simulink model "Vehicle_Model_Controller_Aug13"  (R2021b)
settings: Solver=VariableStepAuto  StartTime=0.0  StopTime=15  FixedStep=0.015  MaxStep=0.015  RelTol=1e-3
model workspace (MAT data in the model file):
  Cx = 10000
  Dx = 2000
  Kp = 10
  understeer_gradient = 0.05
values from neighbouring files (symbols this model uses):
  a = Simulink.Parameter(1.14)    [startup.m]
  A1 = Simulink.Parameter(39.8344)    [startup.m]
  A2 = Simulink.Parameter(813.0780)    [startup.m]
  b = Simulink.Parameter(-0.03291)    [startup.m]
  B1 = Simulink.Parameter(0.000001287)    [startup.m]
  B2 = Simulink.Parameter(-0.002325)    [startup.m]
  B3 = Simulink.Parameter(3.797)    [startup.m]
  c = Simulink.Parameter(-1.14)    [startup.m]
  C1 = Simulink.Parameter(-0.000000002541)    [startup.m]
  C2 = Simulink.Parameter(0.000005279)    [startup.m]
  C3 = Simulink.Parameter(-0.003943)    [startup.m]
  C4 = Simulink.Parameter(3.634)    [startup.m]
  C_param = Simulink.Parameter([0 13757.41 21278.97 26666.02 30253.47 30313.18 30313.18])    [startup.m]
  d = Simulink.Parameter(-1.027)    [startup.m]
  driver_gain = 1    [startup.m]
  FZ_C = Simulink.Parameter([0 204.13 427.04 668.1 895.72 1124.40 1324.40])    [startup.m]
  gr = Simulink.Parameter([6.63043, 6.63043, 7.95652, 7.95652])    [startup.m]
  I = 15    [startup.m]
  inch2mm = Simulink.Parameter(25.4)    [startup.m]
  J_z = Simulink.Parameter(75)    [startup.m]
  k_limit = Simulink.Parameter(3.461)    [startup.m]
  Ku = Simulink.Parameter(0.24 / g.Value)    [startup.m]
  l = Simulink.Parameter([0.7922471, 0.7828529])    [startup.m]
  max_yaw_field = Simulink.Parameter([1.34 1.34 1.34 1.66 1.14 1.24 0.754 0.849 0.85 0.85])    [startup.m]
  min_speed_regen = Simulink.Parameter(85)    [startup.m]
  motor_efficiency = Simulink.Parameter([0.85, 0.85, 0.85, 0.85])    [startup.m]
  motor_limit_power = Simulink.Parameter([15000, 15000, 15000, 15000])    [startup.m]
  motor_limit_torque = Simulink.Parameter([-25, 25])    [startup.m]
  mu_factor = Simulink.Parameter(2/3)    [startup.m]
  P = 1    [startup.m]
  ramp_rate = 1    [startup.m]
  RE = Simulink.Parameter(0.2228169203)    [startup.m]
  s = Simulink.Parameter([0.647895, 0.62102])    [startup.m]
  S1 = Simulink.Parameter(7 * (10^(-5)))    [startup.m]
  S2 = Simulink.Parameter(-0.0038)    [startup.m]
  S3 = Simulink.Parameter(0.6535)    [startup.m]
  S4 = Simulink.Parameter(0.1061)    [startup.m]
  steer_slope = Simulink.Parameter(0.0111)    [startup.m]
  T = 0    [startup.m]
  T2F = Simulink.Parameter(single([29 29 35 35]))    [startup.m]
  tau = Simulink.Parameter(0)    [startup.m]
  time_delay = 0.022    [startup.m]
  V_target = Simulink.Parameter([0 3 6 9 12 15 18 21 25 31])    [startup.m]
undefined symbols (not defined in the file or in its folder): DiscIntNeverNeededParam
libraries: fl_lib x42, nesl_utility x37, sdl_lib x11, slpidlib x1, vehdynlibtire x1, autolibshared x1, autolibdatasheetbattery x1
(part 1 of 4)
settings Model: TunableVars=F_sv,F_x_ij,F_x_ij_max,F_y_fl,F_y_fr,F_y_ij,F_y_rl,F_y_rr,J_z,K_1,K_2,LB,PID,R,T_x_ij,UP,delta,driver_input,err,l,l_f,l_r,linsol,s,s_f,s_r,x,x_1,x_2,x_3,x_4,y,y_1,y_2,y_3,y_4  TunableVarsStorageClass=Auto,Auto,Auto,Auto,Auto,Auto,Auto,Auto,Auto,Auto,Auto,Auto,Auto,Auto,Auto,Auto,Auto,Auto,Auto,Auto,Auto,Auto,Auto,Auto,Auto,Auto,Auto,Auto,Auto,Auto,Auto,Auto,Auto,Auto,Auto,Auto  TunableVarsTypeQualifier=,,,,,,,,,,,,,,,,,,,,,,,,,,,,,,,,,,,  ParameterArgumentNames=understeer_gradient  Creator=True  LastModifiedBy=Inver
settings SolverCC: MaxConsecutiveMinStep=10  AlgebraicLoopSolver=TrustRegion  AutoInsertRateTranBlk=on  MinimalZcImpactIntegration=on
settings DataIOCC: ExternalInput=straight_accel.getElement('driver_input'),straight_accel.getElement('P_A'),straight_accel.getElement('B_A'),straight_accel.getElement('steering_angle'),straight_accel.getElement('wind x'),straight_accel.getElement('wind y'),straight_accel.getElement('wind z'),straight_accel.getElement('batt_temp'),straight_accel.getElement('pressure_front'),straight_accel.getElement('pressure_rear')  LoadExternalInput=on
settings OptimizationCC: DefaultParameterBehavior=Inlined  UseFloatMulNetSlope=on  InlineInvariantSignals=on  BufferReuse=off  EnhancedBackFolding=on  PassReuseOutputArgsThreshold=0  EfficientFloat2IntCast=on  EfficientMapNaN2IntZero=off  OptimizeBlockOrder=speed  DifferentSizesBufferReuse=on
settings DebuggingCC: RTPrefix=warning  SignalInfNanChecking=error  ReadBeforeWriteMsg=DisableAll  WriteAfterWriteMsg=DisableAll  WriteAfterReadMsg=DisableAll  SolverPrmCheckMsg=error  MultiTaskDSMMsg=none  ParameterTunabilityLossMsg=error  SFMachineParentedDataDiag=warning  ArithmeticOperatorsInVariantConditions=warning
settings HardwareCC: TargetBitPerPointer=64  TargetBitPerSizeT=64  TargetBitPerPtrDiffT=64  TargetLongLongMode=on  TargetIntDivRoundTo=Zero  TargetEndianess=LittleEndian  TargetWordSize=64  TargetHWDeviceType=MATLAB Host  ProdEqTarget=off
settings ModelReferenceCC: UpdateModelReferenceTargets=IfOutOfDate
settings SFSimCC: SimCustomHeaderCode="#include \"bigM_v2_func.h\""  SimUserSources=bigM_v2_func.c  SimUserIncludeDirs=$matlabroot$\toolbox\rtw\rtwdemos\EmbeddedCoderOverview\  SFSimEcho=off  CustomCodeUndefinedFunction=UseInterfaceOnly
settings RTWCC: Description=Rapid Simulation Target  SystemTargetFile=rsim.tlc  GenCodeOnly=on  TemplateMakefile=rsim_default_tmf  GenerateReport=on  BuildConfiguration=Faster Runs  LaunchReport=on  CheckMdlBeforeBuild=Warning
settings CodeAppCC: ForceParamTrailComments=on  OperatorAnnotations=on
settings RSimTargetCC: TargetLangStandard=C99 (ISO)
settings ConfigComp: CovScope=ReferencedModels  DVMaxProcessTime=100  DVTestSuiteOptimization=CombinedObjectives (Nonlinear Extended)  DVDetectOutOfBounds=on
settings SimscapeCC: SimscapeLogType=local

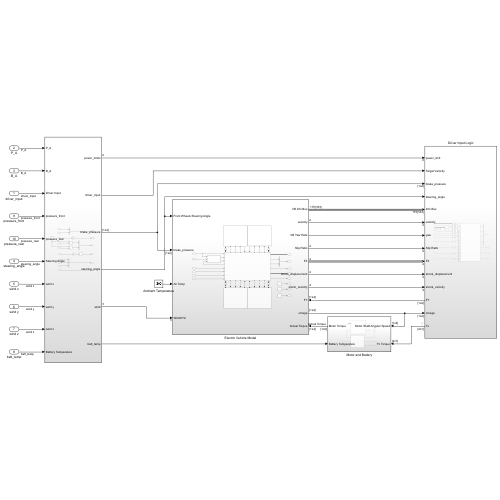
[thumbnail: Simulink's stored preview of the top-level diagram]
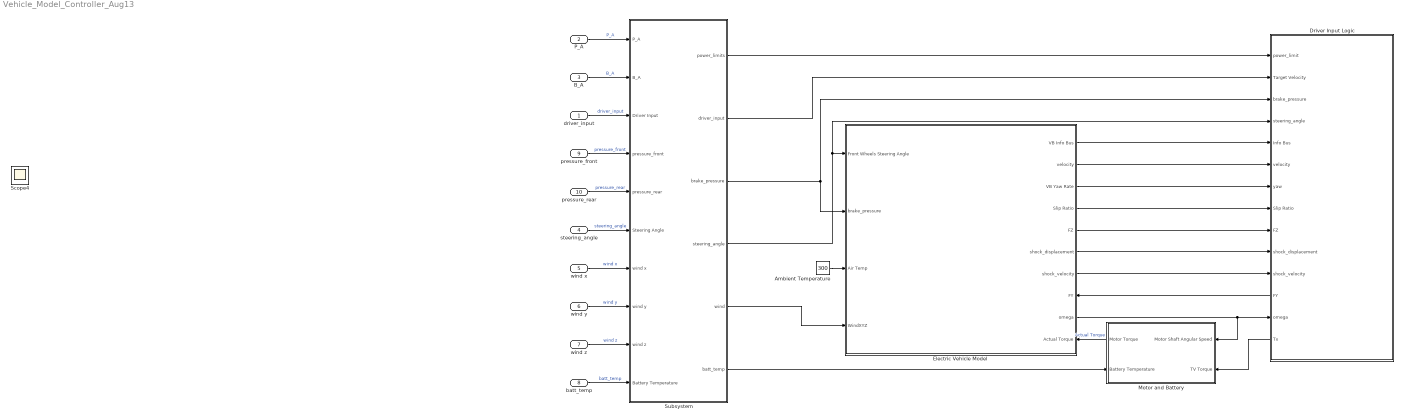
== system Vehicle_Model_Controller_Aug13 ==
  driver_input : Inport  Interpolate=off
  P_A : Inport  Port=2  Interpolate=off
  B_A : Inport  Port=3  Interpolate=off
  steering_angle : Inport  Port=4
  wind x : Inport  Port=5  Interpolate=off
  wind y : Inport  Port=6  Interpolate=off
  wind z : Inport  Port=7  Interpolate=off
  batt_temp : Inport  Port=8  Interpolate=off
  pressure_front : Inport  Port=9  Interpolate=off
  pressure_rear : Inport  Port=10  Interpolate=off
  Ambient Temperature : Constant  Value=300
  Driver Input Logic : Subsystem
      settings: PortSchema="{\"entries\":[{\"content\":{\"sides\":[{\"content\":{\"connectorIds\":[\"In1\",\"In2\",\"In3\",\"In4\",\"In5\",\"In6\",\"In7\",\"In8\",\"In9\",\"In10\",\"In11\",\"Out1\",\"In12\",\"Out2\"]},\"type\":\"ConnectorPlacement.EquallySpacedRectSide\",\"uuid\":\"60aa76ce-4868-40a7-a4fe-105a8e1f1745\"},{\"content\":{\"connectorIds\":[],\"side\":\"RIGHT\"},\"type\":\"ConnectorPlacement.EquallySpacedRectSide\",\"uuid\":\"32a33737-884d-4b24-9f96-3d3edd17fbca\"},{\"content\":{\"connectorIds\":[],\"side\":\"TOP\"},\"type\":\"ConnectorPlacement.EquallySpacedRectSide\",\"uuid\":\"827704d2-5b88-4535-b448-6dd72aa29b4b\"},{\"content\":{\"connectorIds\":[],\"side\":\"BOTTOM\"},\"type\":\"ConnectorPlacement.EquallySpacedRectSide\",\"uuid\":\"278cc67c-48ea-4083-b722-927ef88660f9\"},{\"content\":{\"connectorIds\":[],\"side\":\"HIDDEN\"},\"type\":\"ConnectorPlacement.EquallySpacedRectSide\",\"uuid\":\"0c403b58-0099-4716-b0b3-86e3ff44a502\"}]},\"type\":\"ConnectorPlacement.EquallySpacedConnector\",\"uuid\":\"f0e3ee49-9104-4d68-bbfb-d96c82f46588\"}],\"packageUris\":[\"http://schema.mathworks.com/mf0/Connector/R2020b\"],\"version\":\"1.0\"}"
  Electric Vehicle Model : Subsystem
      settings: PortSchema="{\"entries\":[{\"content\":{\"sides\":[{\"content\":{\"connectorIds\":[\"In1\",\"In2\",\"In3\",\"In4\"]},\"type\":\"ConnectorPlacement.EquallySpacedRectSide\",\"uuid\":\"d948e6fd-2a7c-48d4-af15-7a99a175752d\"},{\"content\":{\"connectorIds\":[\"Out1\",\"Out2\",\"Out3\",\"Out4\",\"Out5\",\"Out6\",\"Out7\",\"In5\",\"Out8\",\"In6\"],\"side\":\"RIGHT\"},\"type\":\"ConnectorPlacement.EquallySpacedRectSide\",\"uuid\":\"1a47e5e8-2455-404d-921d-9ae775b78aa8\"},{\"content\":{\"connectorIds\":[],\"side\":\"TOP\"},\"type\":\"ConnectorPlacement.EquallySpacedRectSide\",\"uuid\":\"f91bd10b-9e07-4da1-95e5-01fed64ff2a2\"},{\"content\":{\"connectorIds\":[],\"side\":\"BOTTOM\"},\"type\":\"ConnectorPlacement.EquallySpacedRectSide\",\"uuid\":\"a21defd9-60a5-4926-b7a0-aedbd24b2311\"},{\"content\":{\"connectorIds\":[],\"side\":\"HIDDEN\"},\"type\":\"ConnectorPlacement.EquallySpacedRectSide\",\"uuid\":\"26c45b26-0233-46e7-86a3-2b3d6a7840e5\"}]},\"type\":\"ConnectorPlacement.EquallySpacedConnector\",\"uuid\":\"a0d97086-54ab-4f92-bc82-b1adaed3f48d\"}],\"packageUris\":[\"http://schema.mathworks.com/mf0/Connector/R2020b\"],\"version\":\"1.0\"}"
  Motor and Battery : Subsystem
      settings: PortSchema="{\"entries\":[{\"content\":{\"sides\":[{\"content\":{\"connectorIds\":[\"Out1\",\"In1\"]},\"type\":\"ConnectorPlacement.EquallySpacedRectSide\",\"uuid\":\"0a1f914b-70eb-46fa-9e3d-552685e5145b\"},{\"content\":{\"connectorIds\":[\"In2\",\"In3\"],\"side\":\"RIGHT\"},\"type\":\"ConnectorPlacement.EquallySpacedRectSide\",\"uuid\":\"3f4913ad-53b1-4c2d-9942-63851d66d84d\"},{\"content\":{\"connectorIds\":[],\"side\":\"TOP\"},\"type\":\"ConnectorPlacement.EquallySpacedRectSide\",\"uuid\":\"355326fa-9c02-45e7-a319-d2a0d6b3d4bd\"},{\"content\":{\"connectorIds\":[],\"side\":\"HIDDEN\"},\"type\":\"ConnectorPlacement.EquallySpacedRectSide\",\"uuid\":\"65af7ff0-f0aa-4be0-a188-dc3dcb8956e6\"}]},\"type\":\"ConnectorPlacement.EquallySpacedConnector\",\"uuid\":\"023a46d9-a637-4c8e-84c1-6893dcef87c2\"}],\"packageUris\":[\"http://schema.mathworks.com/mf0/Connector/R2020b\"],\"version\":\"1.0\"}"
  Subsystem : Subsystem
  Scope4 : Scope
  wires:
  Ambient Temperature/1 -> Electric Vehicle Model/3(Air Temp)
  Electric Vehicle Model/1(VB Info Bus) -> Driver Input Logic/5(Info Bus)
  Electric Vehicle Model/2(velocity) -> Driver Input Logic/6(velocity)
  Electric Vehicle Model/3(VB Yaw Rate) -> Driver Input Logic/7(yaw)
  Driver Input Logic/2(Tx) -> Motor and Battery/3(TV Torque)
  Electric Vehicle Model/4(Slip Ratio) -> Driver Input Logic/8(Slip Ratio)
  Electric Vehicle Model/5(FZ) -> Driver Input Logic/9(FZ)
  Motor and Battery/1(Motor Torque) -> Electric Vehicle Model/6(Actual Torque)  "Actual Torque"
  Electric Vehicle Model/8(omega) -> Motor and Battery/2(Motor Shaft Angular Speed), Driver Input Logic/12(omega)
  Electric Vehicle Model/6(shock_displacement) -> Driver Input Logic/10(shock_displacement)
  Electric Vehicle Model/7(shock_velocity) -> Driver Input Logic/11(shock_velocity)
  Driver Input Logic/1(FY) -> Electric Vehicle Model/5(FY)
  Subsystem/4(steering_angle) -> Driver Input Logic/4(steering_angle), Electric Vehicle Model/1(Front Wheels Steering Angle)
  Subsystem/3(brake_pressure) -> Driver Input Logic/3(brake_pressure), Electric Vehicle Model/2(brake_pressure)
  P_A/1 -> Subsystem/1(P_A)  "P_A"
  B_A/1 -> Subsystem/2(B_A)  "B_A"
  driver_input/1 -> Subsystem/3(Driver Input)  "driver_input"
  pressure_front/1 -> Subsystem/4(pressure_front)  "pressure_front"
  pressure_rear/1 -> Subsystem/5(pressure_rear)  "pressure_rear"
  steering_angle/1 -> Subsystem/6(Steering Angle)  "steering_angle"
  wind x/1 -> Subsystem/7(wind x)  "wind x"
  wind y/1 -> Subsystem/8(wind y)  "wind y"
  wind z/1 -> Subsystem/9(wind z)  "wind z"
  Subsystem/1(power_limits) -> Driver Input Logic/1(power_limit)
  Subsystem/2(driver_input) -> Driver Input Logic/2(Target Velocity)
  Subsystem/5(wind) -> Electric Vehicle Model/4(WindXYZ)
  batt_temp/1 -> Subsystem/10(Battery Temperature)  "batt_temp"
  Subsystem/6(batt_temp) -> Motor and Battery/1(Battery Temperature)

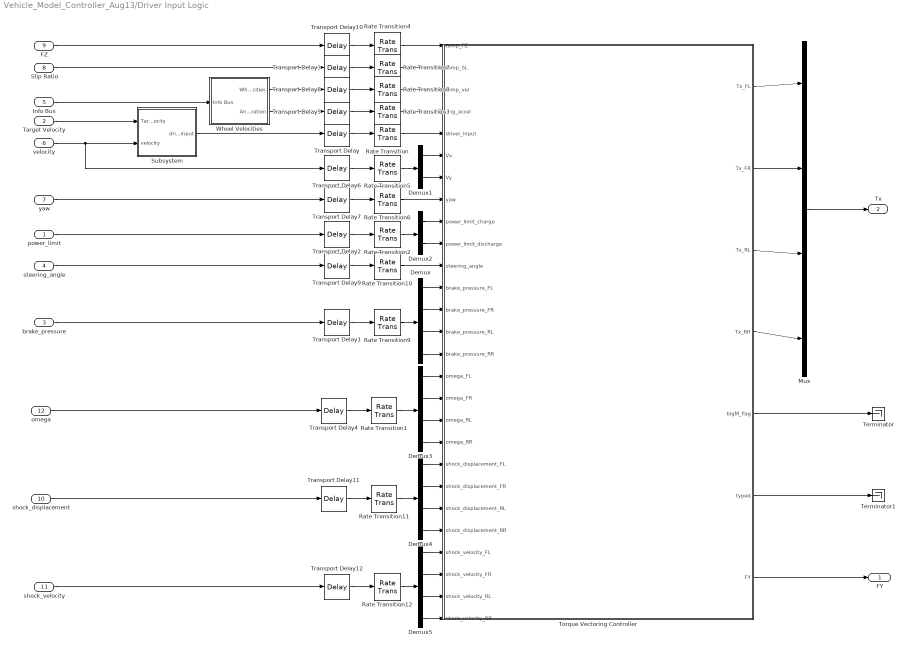
== system Vehicle_Model_Controller_Aug13/Driver Input Logic ==
  power_limit : Inport
  Target Velocity : Inport  Port=2
  brake_pressure : Inport  Port=3  PortDimensions=[1 4]
  steering_angle : Inport  Port=4
  Info Bus : Inport  Port=5
  velocity : Inport  Port=6
  yaw : Inport  Port=7
  Slip Ratio : Inport  Port=8
  FZ : Inport  Port=9
  shock_displacement : Inport  Port=10
  shock_velocity : Inport  Port=11
  omega : Inport  Port=12
  " Wheel Velocities" : Subsystem
  Demux{,3..5} (4 alike) : Demux
  Demux1 : Demux  Outputs=2
  Demux2 : Demux  Outputs=2
  Mux : Mux
  Rate Transition{,1,3,5..6,10..12} (8 alike) : RateTransition  OutPortSampleTime=0.015
  Rate Transition2 : RateTransition  InitialCondition=[0 0]  OutPortSampleTime=0.015
  Rate Transition4 : RateTransition  InitialCondition=[450 450 450 450]  OutPortSampleTime=0.015
  Rate Transition7 : RateTransition  InitialCondition=[0 0 0 0]  OutPortSampleTime=0.015
  Rate Transition8 : RateTransition  InitialCondition=[0 0 0 0 0 0]  OutPortSampleTime=0.015
  Rate Transition9 : RateTransition  InitialCondition=[0 0 0 0]  OutPortSampleTime=0.015
  Subsystem : Subsystem
  Terminator : Terminator
  Terminator1 : Terminator
  Torque Vectoring Controller : Subsystem
  Transport Delay{,4..7,9,11..12} (8 alike) : TransportDelay  DelayTime=time_delay  BufferSize=25000
  Transport Delay1 : TransportDelay  DelayTime=time_delay  InitialOutput=[0 0 0 0]  BufferSize=25000
  Transport Delay10 : TransportDelay  DelayTime=time_delay  InitialOutput=[450 450 450 450]  BufferSize=25000
  Transport Delay2 : TransportDelay  DelayTime=time_delay  InitialOutput=[0 0]  BufferSize=25000
  Transport Delay3 : TransportDelay  DelayTime=time_delay  InitialOutput=[0 0 0 0]  BufferSize=25000
  Transport Delay8 : TransportDelay  DelayTime=time_delay  InitialOutput=[0 0 0 0 0 0]  BufferSize=25000
  FY : Outport
  Tx : Outport  Port=2  PortDimensions=[4 1]
  wires:
  Info Bus/1 -> " Wheel Velocities"/1(Info Bus)
  Transport Delay6/1 -> Rate Transition5/1
  Transport Delay3/1 -> Rate Transition7/1
  Transport Delay2/1 -> Rate Transition2/1
  power_limit/1 -> Transport Delay2/1
  Slip Ratio/1 -> Transport Delay3/1
  Transport Delay7/1 -> Rate Transition6/1
  Transport Delay8/1 -> Rate Transition8/1
  " Wheel Velocities"/1(Wheel Velocities) -> Transport Delay8/1
  Transport Delay10/1 -> Rate Transition4/1
  FZ/1 -> Transport Delay10/1
  Subsystem/1(driver_input) -> Transport Delay/1
  yaw/1 -> Transport Delay7/1
  velocity/1 -> Transport Delay6/1, Subsystem/2(velocity)
  Target Velocity/1 -> Subsystem/1(Target Velocity)
  Rate Transition4/1 -> Torque Vectoring Controller/1(temp_FZ)
  Rate Transition8/1 -> Torque Vectoring Controller/3(temp_vel)
  Rate Transition6/1 -> Torque Vectoring Controller/8(yaw)
  Rate Transition/1 -> Torque Vectoring Controller/5(driver_input)
  Transport Delay1/1 -> Rate Transition9/1
  brake_pressure/1 -> Transport Delay1/1
  Transport Delay9/1 -> Rate Transition10/1
  steering_angle/1 -> Transport Delay9/1
  Rate Transition10/1 -> Torque Vectoring Controller/11(steering_angle)
  Torque Vectoring Controller/1(Tx_FL) -> Mux/1
  Torque Vectoring Controller/2(Tx_FR) -> Mux/2
  Torque Vectoring Controller/3(Tx_RL) -> Mux/3
  Torque Vectoring Controller/4(Tx_RR) -> Mux/4
  Mux/1 -> Tx/1
  Torque Vectoring Controller/5(bigM_flag) -> Terminator/1
  Torque Vectoring Controller/6(typed) -> Terminator1/1
  Rate Transition9/1 -> Demux/1
  Rate Transition7/1 -> Torque Vectoring Controller/2(temp_SL)
  Rate Transition5/1 -> Demux1/1
  Demux1/1 -> Torque Vectoring Controller/6(Vx)
  Demux1/2 -> Torque Vectoring Controller/7(Vy)
  Rate Transition2/1 -> Demux2/1
  Demux2/1 -> Torque Vectoring Controller/9(power_limit_charge)
  Demux2/2 -> Torque Vectoring Controller/10(power_limit_discharge)
  Demux/1 -> Torque Vectoring Controller/12(brake_pressure_FL)
  Transport Delay5/1 -> Rate Transition3/1
  Rate Transition3/1 -> Torque Vectoring Controller/4(ang_accel)
  " Wheel Velocities"/2(Angular Acceleration) -> Transport Delay5/1
  Transport Delay/1 -> Rate Transition/1
  Demux5/4 -> Torque Vectoring Controller/27(shock_velocity_RR)
  Demux5/3 -> Torque Vectoring Controller/26(shock_velocity_RL)
  Demux5/2 -> Torque Vectoring Controller/25(shock_velocity_FR)
  Demux5/1 -> Torque Vectoring Controller/24(shock_velocity_FL)
  Demux4/4 -> Torque Vectoring Controller/23(shock_displacement_RR)
  Demux4/3 -> Torque Vectoring Controller/22(shock_displacement_RL)
  Demux4/2 -> Torque Vectoring Controller/21(shock_displacement_FR)
  Demux4/1 -> Torque Vectoring Controller/20(shock_displacement_FL)
  Demux3/4 -> Torque Vectoring Controller/19(omega_RR)
  Demux3/3 -> Torque Vectoring Controller/18(omega_RL)
  Demux3/2 -> Torque Vectoring Controller/17(omega_FR)
  Demux3/1 -> Torque Vectoring Controller/16(omega_FL)
  Rate Transition12/1 -> Demux5/1
  Rate Transition11/1 -> Demux4/1
  Rate Transition1/1 -> Demux3/1
  Transport Delay4/1 -> Rate Transition1/1
  Transport Delay11/1 -> Rate Transition11/1
  Transport Delay12/1 -> Rate Transition12/1
  omega/1 -> Transport Delay4/1
  shock_displacement/1 -> Transport Delay11/1
  shock_velocity/1 -> Transport Delay12/1
  Torque Vectoring Controller/7(FY) -> FY/1
  Demux/2 -> Torque Vectoring Controller/13(brake_pressure_FR)
  Demux/3 -> Torque Vectoring Controller/14(brake_pressure_RL)
  Demux/4 -> Torque Vectoring Controller/15(brake_pressure_RR)

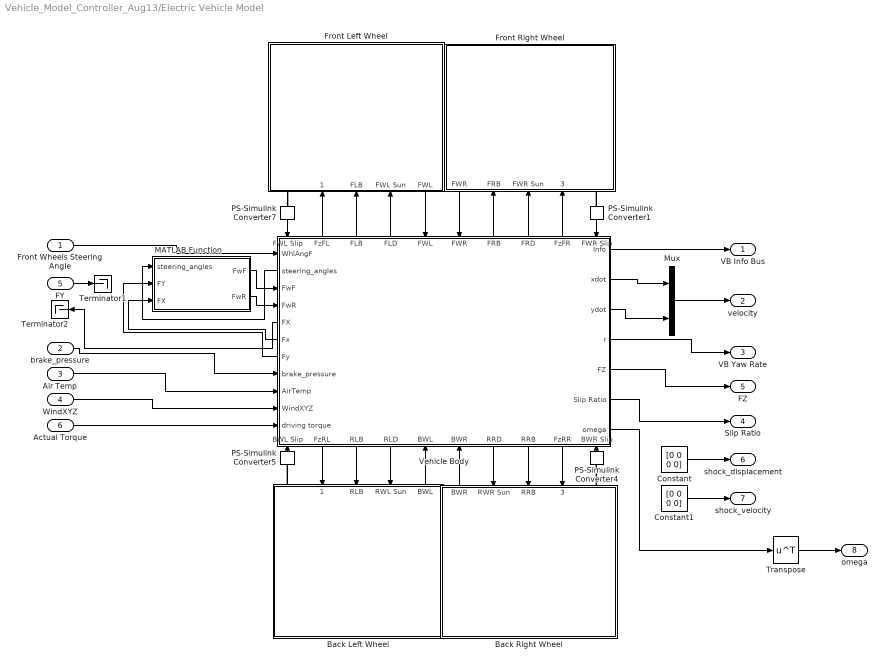
== system Vehicle_Model_Controller_Aug13/Electric Vehicle Model ==
  Front Wheels Steering Angle : Inport
  brake_pressure : Inport  Port=2
  Air Temp : Inport  Port=3
  WindXYZ : Inport  Port=4
  FY : Inport  Port=5
  Actual Torque : Inport  Port=6
  Back Left Wheel : Subsystem
      settings: PortSchema="{\"entries\":[{\"content\":{\"sides\":[{\"content\":{\"connectorIds\":[]},\"type\":\"ConnectorPlacement.EquallySpacedRectSide\",\"uuid\":\"2b71f4a5-a413-4669-bce9-c022c008b37f\"},{\"content\":{\"connectorIds\":[],\"side\":\"RIGHT\"},\"type\":\"ConnectorPlacement.EquallySpacedRectSide\",\"uuid\":\"bc97bf18-1824-4dcb-a7bf-b21d223b914e\"},{\"content\":{\"connectorIds\":[\"LConn1\",\"In1\",\"In2\",\"In3\",\"Out1\"],\"side\":\"TOP\"},\"type\":\"ConnectorPlacement.EquallySpacedRectSide\",\"uuid\":\"45ab5d46-9661-4401-8349-74a293812c9f\"},{\"content\":{\"connectorIds\":[],\"side\":\"HIDDEN\"},\"type\":\"ConnectorPlacement.EquallySpacedRectSide\",\"uuid\":\"98f7b348-3a36-4ee3-a398-c35d25fd5096\"}]},\"type\":\"ConnectorPlacement.EquallySpacedConnector\",\"uuid\":\"08ca7540-1c7d-4720-99bc-9cfb6f12d06d\"}],\"packageUris\":[\"http://schema.mathworks.com/mf0/Connector/R2020b\"],\"version\":\"1.0\"}"
  Back Right Wheel : Subsystem
      settings: PortSchema="{\"entries\":[{\"content\":{\"sides\":[{\"content\":{\"connectorIds\":[]},\"type\":\"ConnectorPlacement.EquallySpacedRectSide\",\"uuid\":\"0dce7c84-f49c-47da-a985-42537e31f80d\"},{\"content\":{\"connectorIds\":[],\"side\":\"RIGHT\"},\"type\":\"ConnectorPlacement.EquallySpacedRectSide\",\"uuid\":\"6a2d686c-11f7-455f-a903-3ea36dc1e6c4\"},{\"content\":{\"connectorIds\":[\"Out1\",\"In1\",\"In2\",\"In3\",\"LConn1\"],\"side\":\"TOP\"},\"type\":\"ConnectorPlacement.EquallySpacedRectSide\",\"uuid\":\"f7c89490-d7ec-4842-8f49-6b07ecd893d9\"},{\"content\":{\"connectorIds\":[],\"side\":\"HIDDEN\"},\"type\":\"ConnectorPlacement.EquallySpacedRectSide\",\"uuid\":\"1095a815-35e8-40c4-8518-dd6454b2f370\"}]},\"type\":\"ConnectorPlacement.EquallySpacedConnector\",\"uuid\":\"2c7105c5-1f43-4c21-98a2-86270cd61bf9\"}],\"packageUris\":[\"http://schema.mathworks.com/mf0/Connector/R2020b\"],\"version\":\"1.0\"}"
  Constant : Constant  Value=[0 0 0 0]
  Constant1 : Constant  Value=[0 0 0 0]
  Front Left Wheel : Subsystem
      settings: PortSchema="{\"entries\":[{\"content\":{\"sides\":[{\"content\":{\"connectorIds\":[]},\"type\":\"ConnectorPlacement.EquallySpacedRectSide\",\"uuid\":\"2b71f4a5-a413-4669-bce9-c022c008b37f\"},{\"content\":{\"connectorIds\":[],\"side\":\"RIGHT\"},\"type\":\"ConnectorPlacement.EquallySpacedRectSide\",\"uuid\":\"bc97bf18-1824-4dcb-a7bf-b21d223b914e\"},{\"content\":{\"connectorIds\":[],\"side\":\"TOP\"},\"type\":\"ConnectorPlacement.EquallySpacedRectSide\",\"uuid\":\"45ab5d46-9661-4401-8349-74a293812c9f\"},{\"content\":{\"connectorIds\":[\"RConn1\",\"In1\",\"In2\",\"In3\",\"Out1\"],\"side\":\"BOTTOM\"},\"type\":\"ConnectorPlacement.EquallySpacedRectSide\",\"uuid\":\"626a829b-c6a7-44fa-8f29-1d2c0438f6d4\"},{\"content\":{\"connectorIds\":[],\"side\":\"HIDDEN\"},\"type\":\"ConnectorPlacement.EquallySpacedRectSide\",\"uuid\":\"98f7b348-3a36-4ee3-a398-c35d25fd5096\"}]},\"type\":\"ConnectorPlacement.EquallySpacedConnector\",\"uuid\":\"08ca7540-1c7d-4720-99bc-9cfb6f12d06d\"}],\"packageUris\":[\"http://schema.mathworks.com/mf0/Connector/R2020b\"],\"version\":\"1.0\"}"
  Front Right Wheel : Subsystem
      settings: PortSchema="{\"entries\":[{\"content\":{\"sides\":[{\"content\":{\"connectorIds\":[]},\"type\":\"ConnectorPlacement.EquallySpacedRectSide\",\"uuid\":\"0dce7c84-f49c-47da-a985-42537e31f80d\"},{\"content\":{\"connectorIds\":[],\"side\":\"RIGHT\"},\"type\":\"ConnectorPlacement.EquallySpacedRectSide\",\"uuid\":\"6a2d686c-11f7-455f-a903-3ea36dc1e6c4\"},{\"content\":{\"connectorIds\":[],\"side\":\"TOP\"},\"type\":\"ConnectorPlacement.EquallySpacedRectSide\",\"uuid\":\"f7c89490-d7ec-4842-8f49-6b07ecd893d9\"},{\"content\":{\"connectorIds\":[\"Out1\",\"In1\",\"In2\",\"In3\",\"RConn1\"],\"side\":\"BOTTOM\"},\"type\":\"ConnectorPlacement.EquallySpacedRectSide\",\"uuid\":\"41036381-c0f5-4b34-b4f9-9bf6c3122150\"},{\"content\":{\"connectorIds\":[],\"side\":\"HIDDEN\"},\"type\":\"ConnectorPlacement.EquallySpacedRectSide\",\"uuid\":\"1095a815-35e8-40c4-8518-dd6454b2f370\"}]},\"type\":\"ConnectorPlacement.EquallySpacedConnector\",\"uuid\":\"2c7105c5-1f43-4c21-98a2-86270cd61bf9\"}],\"packageUris\":[\"http://schema.mathworks.com/mf0/Connector/R2020b\"],\"version\":\"1.0\"}"
  MATLAB Function : MATLAB Function  TreatAsAtomicUnit=on  SystemSampleTime=0.015
  Mux : Mux  Inputs=2
  PS-Simulink Converter{1,4..5,7} (4 alike) : nesl_utility/PS-Simulink Converter  PhysicalDomain=network_engine_domain  SubClassName=ps_output  LeftPortType=input  RightPortType=output  PseudoPeriodic=off  Frequencies=[]  Unit=inherit  AffineConversion=off
      settings: SourceProductBaseCode=PW,SS
  Terminator1 : Terminator
  Terminator2 : Terminator
  Transpose : Math  Operator=transpose  SaturateOnIntegerOverflow=on
  Vehicle Body : Subsystem
      settings: PortSchema="{\"entries\":[{\"content\":{\"sides\":[{\"content\":{\"connectorIds\":[\"In1\",\"Out20\",\"In2\",\"In3\",\"Out21\",\"Out22\",\"Out23\",\"In4\",\"In5\",\"In6\",\"In7\"]},\"type\":\"ConnectorPlacement.EquallySpacedRectSide\",\"uuid\":\"603222f6-0091-4ad0-bf19-39b4be84e01e\"},{\"content\":{\"connectorIds\":[\"Out1\",\"Out2\",\"Out3\",\"Out4\",\"Out5\",\"Out6\",\"Out7\"],\"side\":\"RIGHT\"},\"type\":\"ConnectorPlacement.EquallySpacedRectSide\",\"uuid\":\"c4db7259-b5a3-4868-8718-dda29d48254f\"},{\"content\":{\"connectorIds\":[\"In8\",\"Out14\",\"Out15\",\"Out16\",\"In9\",\"In10\",\"Out17\",\"Out18\",\"Out19\",\"In11\"],\"side\":\"TOP\"},\"type\":\"ConnectorPlacement.EquallySpacedRectSide\",\"uuid\":\"a713a325-471a-4f93-96c3-fb024f273799\"},{\"content\":{\"connectorIds\":[\"In12\",\"Out8\",\"Out9\",\"Out10\",\"In13\",\"In14\",\"Out11\",\"Out12\",\"Out13\",\"In15\"],\"side\":\"BOTTOM\"},\"type\":\"ConnectorPlacement.EquallySpacedRectSide\",\"uuid\":\"12db6ab3-ce51-4037-9ece-8ccfa03e22af\"},{\"content\":{\"connectorIds\":[],\"side\":\"HIDDEN\"},\"type\":\"ConnectorPlacement.EquallySpacedRectSide\",\"uuid\":\"dd051903-611f-41d3-87ac-1430d6d99127\"}]},\"type\":\"ConnectorPlacement.EquallySpacedConnector\",\"uuid\":\"5fd2346c-a877-48e3-8a05-bb1d13d3d04b\"}],\"packageUris\":[\"http://schema.mathworks.com/mf0/Connector/R2020b\"],\"version\":\"1.0\"}"
  VB Info Bus : Outport
  velocity : Outport  Port=2
  VB Yaw Rate : Outport  Port=3
  Slip Ratio : Outport  Port=4
  FZ : Outport  Port=5
  shock_displacement : Outport  Port=6
  shock_velocity : Outport  Port=7
  omega : Outport  Port=8  PortDimensions=[1 4]
  wires:
  Vehicle Body/14(FzFL) -> Front Left Wheel/1(FWL Normal)
  PS-Simulink Converter5/1 -> Vehicle Body/12(BWL Slip)
  Vehicle Body/4(r) -> VB Yaw Rate/1
  PS-Simulink Converter4/1 -> Vehicle Body/15(BWR Slip)
  Vehicle Body/8(FzRL) -> Back Left Wheel/1(RWL Normal)
  Vehicle Body/13(FzRR) -> Back Right Wheel/3(BWR Normal)
  Air Temp/1 -> Vehicle Body/5(AirTemp)
  WindXYZ/1 -> Vehicle Body/6(WindXYZ)
  Vehicle Body/1(Info) -> VB Info Bus/1
  Vehicle Body/19(FzFR) -> Front Right Wheel/3(FWR Normal)
  Front Wheels Steering Angle/1 -> Vehicle Body/1(WhlAngF)
  Vehicle Body/16(FLD) -> Front Left Wheel/3(FWL Sun)
  Vehicle Body/18(FRD) -> Front Right Wheel/2(FWR Sun)
  Vehicle Body/15(FLB) -> Front Left Wheel/2(FLB)
  Vehicle Body/17(FRB) -> Front Right Wheel/1(FRB)
  PS-Simulink Converter7/1 -> Vehicle Body/8(FWL Slip)
  PS-Simulink Converter1/1 -> Vehicle Body/11(FWR Slip)
  Vehicle Body/5(FZ) -> FZ/1
  MATLAB Function/2(FwR) -> Vehicle Body/3(FwR)
  MATLAB Function/1(FwF) -> Vehicle Body/2(FwF)
  Vehicle Body/9(RLB) -> Back Left Wheel/2(RLB)
  Vehicle Body/12(RRB) -> Back Right Wheel/2(RRB)
  Vehicle Body/10(RLD) -> Back Left Wheel/3(RWL Sun)
  Vehicle Body/11(RRD) -> Back Right Wheel/1(RWR Sun)
  Back Right Wheel/1(BWR) -> Vehicle Body/14(BWR)
  Back Left Wheel/1(BWL) -> Vehicle Body/13(BWL)
  Front Left Wheel/1(FWL) -> Vehicle Body/9(FWL)
  Front Right Wheel/1(FWR) -> Vehicle Body/10(FWR)
  Actual Torque/1 -> Vehicle Body/7(driving torque)
  Vehicle Body/6(Slip Ratio) -> Slip Ratio/1
  Vehicle Body/2(xdot) -> Mux/1
  Vehicle Body/3(ydot) -> Mux/2
  Mux/1 -> velocity/1
  brake_pressure/1 -> Vehicle Body/4(brake_pressure)
  Constant1/1 -> shock_velocity/1
  Constant/1 -> shock_displacement/1
  Vehicle Body/23(Fy) -> MATLAB Function/2(FY)
  Vehicle Body/22(Fx) -> MATLAB Function/3(FX)
  FY/1 -> Terminator1/1
  Vehicle Body/21(FX) -> Terminator2/1
  Transpose/1 -> omega/1
  Vehicle Body/7(omega) -> Transpose/1
  Vehicle Body/20(steering_angles) -> MATLAB Function/1(steering_angles)
  connections:
  Front Left Wheel/RConn1 -- PS-Simulink Converter7/LConn1
  Back Right Wheel/LConn1 -- PS-Simulink Converter4/LConn1
  Back Left Wheel/LConn1 -- PS-Simulink Converter5/LConn1
  PS-Simulink Converter1/LConn1 -- Front Right Wheel/RConn1

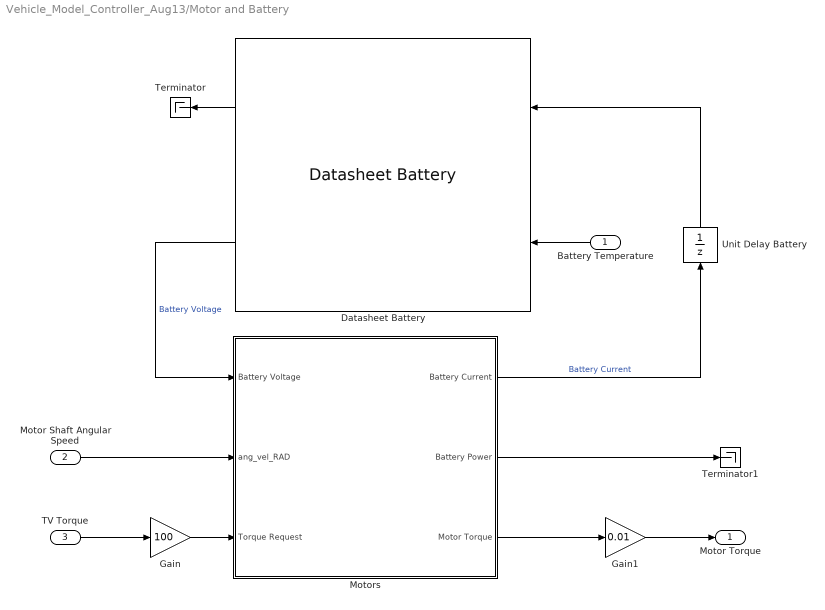
== system Vehicle_Model_Controller_Aug13/Motor and Battery ==
  Battery Temperature : Inport
  Motor Shaft Angular Speed : Inport  Port=2
  TV Torque : Inport  Port=3
  Datasheet Battery : autolibdatasheetbattery/Datasheet Battery  CapacityCtrl=Parameter  OutputVlt=Unfiltered  BattChargeMax=32.5  Em=[2.8 3.228 3.284 3.361 3.408 3.427 3.472 3.477 3.493 3.504 3.516 3.528 3.537 3.545 3.555 3.561 3.566 3.576 3.587 3.589 3.594 3.6 3.608 3.61 3.616 3.619 3.626 3.632 3.637 3.64 3.645 3.646 3.652 3.655 3.658 3.661 3.664 3.668 3.673 3.678 3.68 3.681 3.686 3.692 3.699 3.702 3.705 3.71 3.717 3.723 3.728 3.733 3.735 3.742 3.749 3.755 3.761 3.768 3.773 3.78 3.791 3.798 3.798 3.814 3.818 3.825 3.841 3.846 3.855 3.863 3.877 3.885 3.894 3.907 3.919 3.926 3.935 3.944 3.954 3.964 3.974 3.988 3.998 4.014 4.029 4.034 4.047 4.065 4.074 4.086 4.097 4.131 4.126 4.138 4.15 4.18 4.174 4.187 4.207 4.231 4.221]  CapLUTBp=[0 0.01 0.02 0.03 0.04 0.05 0.06 0.07 0.08 0.09 0.1 0.11 0.12 0.13 0.14 0.15 0.16 0.17 0.18 0.19 0.2 0.21 0.22 0.23 0.24 0.25 0.26 0.27 0.28 0.29 0.3 0.31 0.32 0.33 0.34 0.35 0.36 0.37 0.38 0.39 0.4 0.41 0.42 0.43 0.44 0.45 0.46 0.47 0.48 0.49 0.5 0.51 0.52 0.53 0.54 0.55 0.56 0.57 0.58 0.59 0.6 0.61 0.62 0.63 0.64 0.65 0.66 0.67 0.68 0.69 0.7 0.71 0.72 0.73 0.74 0.75 0.76 0.77 0.78 0.79 0.8 0.81 0.82 0.83 0.84 0.85 0.86 0.87 0.88 0.89 0.9 0.91 0.92 0.93 0.94 0.95 0.96 0.97 0.98 0.99 1]  RInt=[0.008846 0.009319 0.009027 0.00847 0.01032 0.01314;0.006389 0.006554 0.005553 0.005525 0.006043 0.007805;0.004364 0.004101 0.00406 0.003452 0.003846 0.004517;0.002031 0.002563 0.002532 0.00246 0.002716 0.003047;0.001443 0.001825 0.001795 0.001778 0.001924 0.002234;0.0005603 0.0007192 0.0006887 0.0007557 0.0007355 0.001014;0.001028 0.001338 0.001 0.001536 0.001546 0.002789]  BattTempBp=[243.1 253.1 263.1 273.1 283.1 298.1 313.1]  CapSOCBp=[0 0.2 0.4 0.6 0.8 1]  Ns=81  Np=2  BattCapInit=26  Tc=1/1000  Vinit=4.221  RefBlkName='autolibdatasheetbattery/Datasheet Battery'
      settings: SourceProductBaseCode=PW
  Gain : Gain  Gain=100
  Gain1 : Gain  Gain=0.01
  Motors : Subsystem
  Terminator : Terminator
  Terminator1 : Terminator
  Unit Delay Battery : UnitDelay  SampleTime=-1  HasFrameUpgradeWarning=on
  Motor Torque : Outport
  wires:
  Datasheet Battery/1 -> Terminator/1
  Battery Temperature/1 -> Datasheet Battery/2
  Unit Delay Battery/1 -> Datasheet Battery/1
  Motors/1(Battery Current) -> Unit Delay Battery/1  "Battery Current"
  Gain/1 -> Motors/3(Torque Request)
  Gain1/1 -> Motor Torque/1
  Motors/3(Motor Torque) -> Gain1/1
  Motors/2(Battery Power) -> Terminator1/1
  Datasheet Battery/2 -> Motors/1(Battery Voltage)  "Battery Voltage"
  TV Torque/1 -> Gain/1
  Motor Shaft Angular Speed/1 -> Motors/2(ang_vel_RAD)

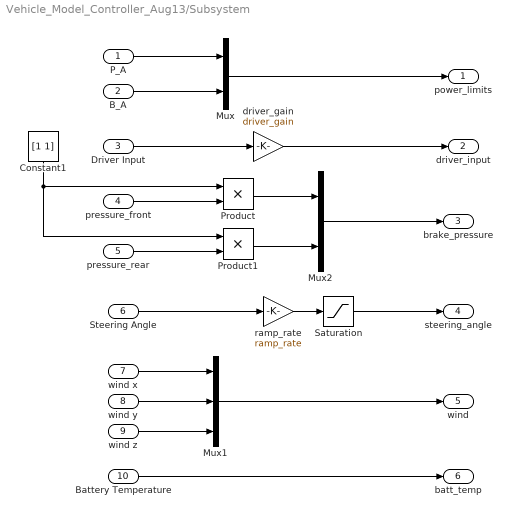
== system Vehicle_Model_Controller_Aug13/Subsystem ==
  P_A : Inport
  B_A : Inport  Port=2
  Driver Input : Inport  Port=3
  pressure_front : Inport  Port=4
  pressure_rear : Inport  Port=5
  Steering Angle : Inport  Port=6
  wind x : Inport  Port=7
  wind y : Inport  Port=8
  wind z : Inport  Port=9
  Battery Temperature : Inport  Port=10
  Constant1 : Constant  Value=[1 1]  VectorParams1D=off
  Mux : Mux  Inputs=2
  Mux1 : Mux  Inputs=3
  Mux2 : Mux  Inputs=2
  Product : Product
  Product1 : Product
  Saturation : Saturate  UpperLimit=30  LowerLimit=-30
  driver_gain : Gain  Gain=driver_gain
  ramp_rate : Gain  Gain=ramp_rate
  power_limits : Outport
  driver_input : Outport  Port=2
  brake_pressure : Outport  Port=3
  steering_angle : Outport  Port=4
  wind : Outport  Port=5
  batt_temp : Outport  Port=6
  wires:
  ramp_rate/1 -> Saturation/1
  wind x/1 -> Mux1/1
  wind z/1 -> Mux1/3
  wind y/1 -> Mux1/2
  Steering Angle/1 -> ramp_rate/1
  Driver Input/1 -> driver_gain/1
  driver_gain/1 -> driver_input/1
  Mux/1 -> power_limits/1
  P_A/1 -> Mux/1
  B_A/1 -> Mux/2
  Saturation/1 -> steering_angle/1
  Mux1/1 -> wind/1
  pressure_front/1 -> Product/2
  Battery Temperature/1 -> batt_temp/1
  Product/1 -> Mux2/1
  Product1/1 -> Mux2/2
  Mux2/1 -> brake_pressure/1
  Constant1/1 -> Product1/1, Product/1
  pressure_rear/1 -> Product1/2

== system Vehicle_Model_Controller_Aug13/Driver Input Logic/ Wheel Velocities ==
  Info Bus : Inport
  Bus Selector1 : BusSelector  OutputSignals=BdyFrm.FrntAxl.Lft.Vel.xdot,BdyFrm.FrntAxl.Lft.Vel.ydot,BdyFrm.FrntAxl.Rght.Vel.xdot,BdyFrm.FrntAxl.Rght.Vel.ydot,BdyFrm.RearAxl.Lft.Vel.xdot,BdyFrm.RearAxl.Rght.Vel.xdot,BdyFrm.Cg.AngAcc.rdot
  Mux : Mux  Inputs=6
  Wheel Velocities : Outport
  Angular Acceleration : Outport  Port=2
  wires:
  Mux/1 -> Wheel Velocities/1
  Bus Selector1/4 -> Mux/4  "<ydot>"
  Bus Selector1/2 -> Mux/2  "<ydot>"
  Bus Selector1/6 -> Mux/6  "<xdot>"
  Bus Selector1/5 -> Mux/5  "<xdot>"
  Bus Selector1/3 -> Mux/3  "<xdot>"
  Bus Selector1/1 -> Mux/1  "<xdot>"
  Info Bus/1 -> Bus Selector1/1
  Bus Selector1/7 -> Angular Acceleration/1  "<rdot>"

== system Vehicle_Model_Controller_Aug13/Driver Input Logic/Subsystem ==
  Target Velocity : Inport
  velocity : Inport  Port=2
  PID Controller : slpidlib/PID Controller  Controller=PID  Form=Parallel  TimeDomain=Discrete-time  UseExternalTs=off  SampleTime=-1  IntegratorMethod=Forward Euler  FilterMethod=Forward Euler  ControllerParametersSource=internal  P=0.2  I=0.2  D=0  UseFilter=on  N=100  TunerSelectOption=Transfer Function Based (PID Tuner App)  InitialConditionSource=internal  InitialConditionForIntegrator=0  InitialConditionForFilter=0  DifferentiatorICPrevScaledInput=0  ExternalReset=none  TrackingMode=off  Kt=1  LimitOutput=on  SatLimitsSource=internal  UpperSaturationLimit=1  LowerSaturationLimit=-1  LinearizeAsGain=on  AntiWindupMode=clamping  Kb=1  POutMin=[]  POutMax=[]  IOutMin=[]  IOutMax=[]  DOutMin=[]  DOutMax=[]  NOutMin=[]  NOutMax=[]  SumOutMin=[]  SumOutMax=[]  SaturationOutMin=[]  SaturationOutMax=[]  PParamMin=[]  PParamMax=[]  IParamMin=[]  IParamMax=[]  DParamMin=[]  DParamMax=[]  NParamMin=[]  NParamMax=[]  KbParamMin=[]  KbParamMax=[]  KtParamMin=[]  KtParamMax=[]  KbOutMin=[]  KbOutMax=[]  KtOutMin=[]  KtOutMax=[]  IntegratorOutMin=[]  IntegratorOutMax=[]  FilterOutMin=[]  FilterOutMax=[]  SumI1OutMin=[]  SumI1OutMax=[]  SumI2OutMin=[]  SumI2OutMax=[]  SumI3OutMin=[]  SumI3OutMax=[]  SumI4OutMin=[]  SumI4OutMax=[]  SumDOutMin=[]  SumDOutMax=[]  DifferentiatorOutMin=[]  DifferentiatorOutMax=[]  FilterDiffOutCoefMin=[]  FilterDiffOutCoefMax=[]  ReciprocalOutMin=[]  ReciprocalOutMax=[]  SumDenOutMin=[]  SumDenOutMax=[]  SumNumOutMin=[]  SumNumOutMax=[]  DivideOutMin=[]  DivideOutMax=[]  UdiffTsProdOutMin=[]  UdiffTsProdOutMax=[]  NTsProdOutMin=[]  NTsProdOutMax=[]  UintegralTsProdOutMin=[]  UintegralTsProdOutMax=[]  UngainTsProdOutMin=[]  UngainTsProdOutMax=[]  IntegratorContinuousStateAttributes=''  IntegratorStateMustResolveToSignalObject=off  IntegratorRTWStateStorageClass=Auto  FilterContinuousStateAttributes=''  FilterStateMustResolveToSignalObject=off  FilterRTWStateStorageClass=Auto  ParallelPVariant=InternalParameters  IdealPVariant=Disabled  IVariant=InternalParameters  DVariant=InternalParameters  IntegratorVariant=Discrete  SatVariant=Enabled  AWVariant=DiscClampingParallel  PCopyVariant=Disabled  TRVariant=Disabled  FdbkBlocksVariant=Forward  IdealPFdbkVariant=Disabled  SatFdbkVariant=Disabled  DerivativeFilterVariant=ForwardEulerFilter  NVariant=InternalParameters  NCopyVariant=Disabled  FilterICVariant=InternalICsFilter  IntegratorICVariant=InternalICs  ExternalResetVariant=Disabled  TRSumVariant=Passthrough  SumFdbkVariant=Disabled  SumVariant=Sum_PID  TsampFilterVariant=InternalTs  TsampNgainVariant=Passthrough  TsampIntegralVariant=Passthrough  ExternalSaturationOutDataTypeStr=Inherit: Same as second input
  Sqrt : Sqrt  SaturateOnIntegerOverflow=on
  Square : Math  Operator=square  SaturateOnIntegerOverflow=on
  Sum : Sum  Inputs=+
  Sum1 : Sum  Inputs=+-
  driver_input : Outport
  wires:
  Target Velocity/1 -> Sum1/1
  Sum1/1 -> PID Controller/1
  Sqrt/1 -> Sum1/2
  Square/1 -> Sum/1
  Sum/1 -> Sqrt/1
  velocity/1 -> Square/1
  PID Controller/1 -> driver_input/1

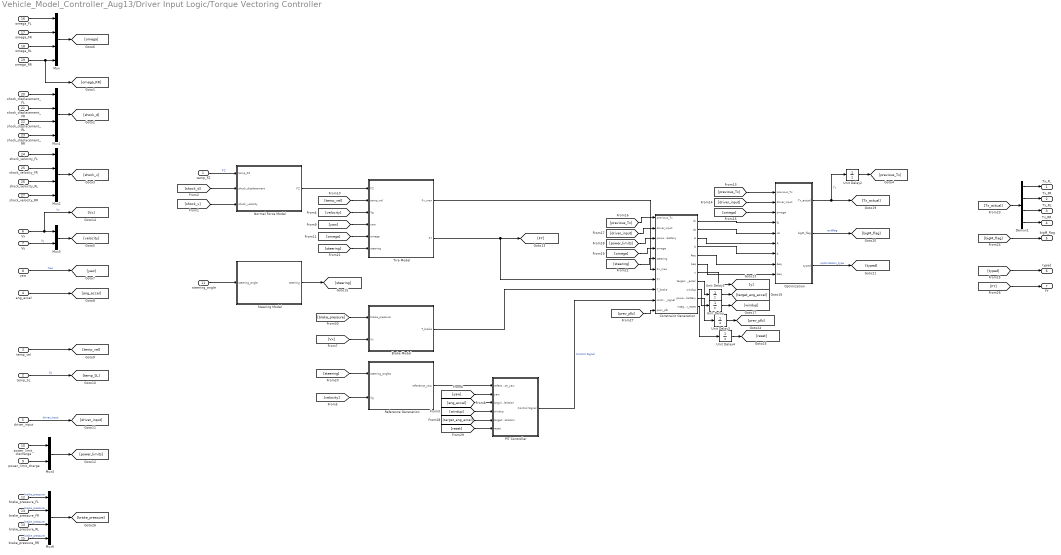
== system Vehicle_Model_Controller_Aug13/Driver Input Logic/Torque Vectoring Controller ==
  temp_FZ : Inport
  temp_SL : Inport  Port=2
  temp_vel : Inport  Port=3
  ang_accel : Inport  Port=4
  driver_input : Inport  Port=5
  Vx : Inport  Port=6
  Vy : Inport  Port=7
  yaw : Inport  Port=8
  power_limit_charge : Inport  Port=9
  power_limit_discharge : Inport  Port=10
  steering_angle : Inport  Port=11
  brake_pressure_FL : Inport  Port=12  PortDimensions=1
  brake_pressure_FR : Inport  Port=13  PortDimensions=1
  brake_pressure_RL : Inport  Port=14  PortDimensions=1
  brake_pressure_RR : Inport  Port=15  PortDimensions=1
  omega_FL : Inport  Port=16
  omega_FR : Inport  Port=17
  omega_RL : Inport  Port=18
  omega_RR : Inport  Port=19  PortDimensions=1
  shock_displacement_FL : Inport  Port=20
  shock_displacement_FR : Inport  Port=21
  shock_displacement_RL : Inport  Port=22
  shock_displacement_RR : Inport  Port=23
  shock_velocity_FL : Inport  Port=24
  shock_velocity_FR : Inport  Port=25
  shock_velocity_RL : Inport  Port=26
  shock_velocity_RR : Inport  Port=27
  Brake Model : MATLAB Function  TreatAsAtomicUnit=on
  Constraint Generation : MATLAB Function  TreatAsAtomicUnit=on
  Demux1 : Demux
  Mux{,1..2,6} (4 alike) : Mux
  Mux3 : Mux  Inputs=2
  Mux4 : Mux  Inputs=2
  Normal Force Model : MATLAB Function  TreatAsAtomicUnit=on
  "Optimization " : MATLAB Function  TreatAsAtomicUnit=on
  PIT Controller : Subsystem
  Reference Generation : MATLAB Function  TreatAsAtomicUnit=on
  Steering Model : MATLAB Function  TreatAsAtomicUnit=on
  Tire Model : MATLAB Function  TreatAsAtomicUnit=on
  Unit Delay{,1..4} (5 alike) : UnitDelay  SampleTime=-1  HasFrameUpgradeWarning=on
  Tx_FL : Outport
  Tx_FR : Outport  Port=2
  Tx_RL : Outport  Port=3
  Tx_RR : Outport  Port=4
  bigM_flag : Outport  Port=5
  typed : Outport  Port=6
  FY : Outport  Port=7
  wires:
  temp_FZ/1 -> Normal Force Model/1(temp_FZ)  "FZ"
  steering_angle/1 -> Steering Model/1(steering_angle)
  Normal Force Model/1(FZ) -> Tire Model/1(FZ)
  [Vx] -> Brake Model/2(Vx)
  omega_FL/1 -> Mux/1
  omega_FR/1 -> Mux/2
  omega_RL/1 -> Mux/3
  omega_RR/1 -> [omega_RR], Mux/4
  shock_displacement_FL/1 -> Mux1/1
  shock_displacement_FR/1 -> Mux1/2
  shock_displacement_RL/1 -> Mux1/3
  shock_displacement_RR/1 -> Mux1/4
  shock_velocity_FL/1 -> Mux2/1
  shock_velocity_FR/1 -> Mux2/2
  shock_velocity_RL/1 -> Mux2/3
  shock_velocity_RR/1 -> Mux2/4
  Mux/1 -> [omega]
  Mux1/1 -> [shock_d]
  Mux2/1 -> [shock_v]
  [shock_v] -> Normal Force Model/3(shock_velocity)
  [shock_d] -> Normal Force Model/2(shock_displacement)
  Vy/1 -> Mux3/2  "Vy"
  Vx/1 -> [Vx], Mux3/1  "Vx"
  Mux3/1 -> [velocity]
  [velocity] -> Reference Generation/2(Vg)
  Reference Generation/1(reference_yaw) -> PIT Controller/1(reference_yaw)
  yaw/1 -> [yaw]  "Yaw"
  [yaw] -> PIT Controller/2(yaw)
  ang_accel/1 -> [ang_accel]
  [ang_accel] -> PIT Controller/3(Angular Acceleration)
  [windup] -> PIT Controller/4(windup)
  [velocity] -> Tire Model/3(Vg)
  [yaw] -> Tire Model/4(yaw)
  [temp_vel] -> Tire Model/2(temp_vel)
  temp_vel/1 -> [temp_vel]
  [omega] -> Tire Model/5(omega)
  temp_SL/1 -> [temp_SL]  "SL"
  [omega] -> "Optimization "/3(omega)
  driver_input/1 -> [driver_input]  "driver_input"
  power_limit_discharge/1 -> Mux4/1
  power_limit_charge/1 -> Mux4/2
  Mux4/1 -> [power_limits]
  [driver_input] -> "Optimization "/2(driver_input)
  [previous_Tx] -> "Optimization "/1(previous_Tx)
  [previous_Tx] -> Constraint Generation/1(previous_Tx)
  [driver_input] -> Constraint Generation/2(driver_input)
  [power_limits] -> Constraint Generation/3(power_limits_battery)
  Tire Model/1(Fx_max) -> Constraint Generation/6(Fx_max)
  Tire Model/2(FY) -> [FY], Constraint Generation/7(FY)
  PIT Controller/1(Control Signal) -> Constraint Generation/9(control_signal)  "Control Signal"
  Brake Model/1(T_brake) -> Constraint Generation/8(T_brake)
  [omega] -> Constraint Generation/4(omega)
  Constraint Generation/1(lb) -> "Optimization "/4(lb)
  Constraint Generation/2(ub) -> "Optimization "/5(ub)
  Constraint Generation/3(A) -> "Optimization "/6(A)
  Constraint Generation/4(b) -> "Optimization "/7(b)
  Constraint Generation/5(Aeq) -> "Optimization "/8(Aeq)
  Constraint Generation/6(beq) -> "Optimization "/9(beq)
  Steering Model/1(steering) -> [steering]
  [steering] -> Reference Generation/1(steering_angles)
  [steering] -> Tire Model/6(steering)
  [steering] -> Constraint Generation/5(steering)
  Demux1/1 -> Tx_FL/1
  Demux1/4 -> Tx_RR/1
  Demux1/3 -> Tx_RL/1
  Demux1/2 -> Tx_FR/1
  "Optimization "/1(Tx_actual) -> [Tx_actual], Unit Delay2/1  "Tx"
  "Optimization "/2(bigM_flag) -> [bigM_flag]  "exitflag"
  "Optimization "/3(typed) -> [typed]  "optimization_type"
  [Tx_actual] -> Demux1/1
  [bigM_flag] -> bigM_flag/1
  [typed] -> typed/1
  [target_ang_accel] -> PIT Controller/5(target_angular_acceleration)
  Unit Delay/1 -> [windup]
  Constraint Generation/9(windup) -> Unit Delay/1
  Unit Delay1/1 -> [target_ang_accel]
  Constraint Generation/8(target_ang_accel) -> Unit Delay1/1
  Unit Delay2/1 -> [previous_Tx]
  [FY] -> FY/1
  Constraint Generation/7(y) -> [y]
  Unit Delay3/1 -> [prev_plb]
  Constraint Generation/10(power_limit_battery) -> Unit Delay3/1
  Constraint Generation/11(integrator_reset) -> Unit Delay4/1
  Unit Delay4/1 -> [reset]
  [prev_plb] -> Constraint Generation/10(prev_plb)
  [reset] -> PIT Controller/6(reset)
  brake_pressure_FL/1 -> Mux6/1  "brake_pressure"
  brake_pressure_FR/1 -> Mux6/2  "brake_pressure"
  brake_pressure_RL/1 -> Mux6/3  "brake_pressure"
  brake_pressure_RR/1 -> Mux6/4  "brake_pressure"
  Mux6/1 -> [brake_pressure]
  [brake_pressure] -> Brake Model/1(brake_pressure)
